simulink model "Demo_TollSystem_cs"  (R2014b)
settings: Solver=FixedStepDiscrete  StartTime=0.0  StopTime=13  FixedStep=1/20  RelTol=1e-3
PreLoadFcn:
  | mbxruntime.callbacks.PreLoadFcn(bdroot);
  | check_NUTS_defined
  | model_closed = 0;
  | assignin('base',['model_closed_' bdroot],false);
PostLoadFcn:
  | mbxruntime.callbacks.PostLoadFcn(bdroot);
InitFcn:
  | mbxruntime.callbacks.InitFcn(bdroot);
StartFcn:
  | mbxruntime.callbacks.StartFcn(bdroot);
  | 
  | open_system([bdroot '/Scope Plot']);
StopFcn:
  | mbxruntime.callbacks.StopFcn(bdroot);
model workspace: external: MAT-File .\Demo_TollSystem_cs_hws.mat (data not in the file)
undefined symbols (not defined in the file): Demo_TollSystem_cs_acfd828c7254e63e, Demo_TollSystem_cs_Mazda_RX8_1_Path_pathUniqueID
libraries: simulink x8, PreScanUsefulBlocks x4
(part 1 of 3)
CloseFcn:
  | mbxruntime.callbacks.CloseFcn(bdroot);
  | evalin('base',['clear model_closed_' bdroot]);
  | model_closed = 1;
settings Model: Creator=PRESCAN  LastModifiedBy=jenkins
settings DataIOCC: SignalLoggingSaveFormat=ModelDataLogs
settings OptimizationCC: InlineParams=on  ExpressionDepthLimit=2147483647  InitFltsAndDblsToZero=on
settings DebuggingCC: SaveWithParameterizedLinksMsg=none  UnderspecifiedInitializationDetection=Classic  MergeDetectMultiDrivingBlocksExec=none  SignalResolutionControl=TryResolveAllWithWarning  SolverPrmCheckMsg=none  MultiTaskDSMMsg=warning  MultiTaskCondExecSysMsg=none  FcnCallInpInsideContextMsg=UseLocalSettings  StateNameClashWarn=warning
settings ModelReferenceCC: UpdateModelReferenceTargets=IfOutOfDate
settings SFSimCC: SimParseCustomCode=off
settings SFSimCC: SimCustomHeaderCode=|
  | #include "prescan.h"
  | #include "prescan_platform.h"
settings RTWCC: IncludeERTFirstTime=on
settings GRTTargetCC: TargetFcnLib=ansi_tfl_tmw.mat  CombineOutputUpdateFcns=off  GRTInterface=on

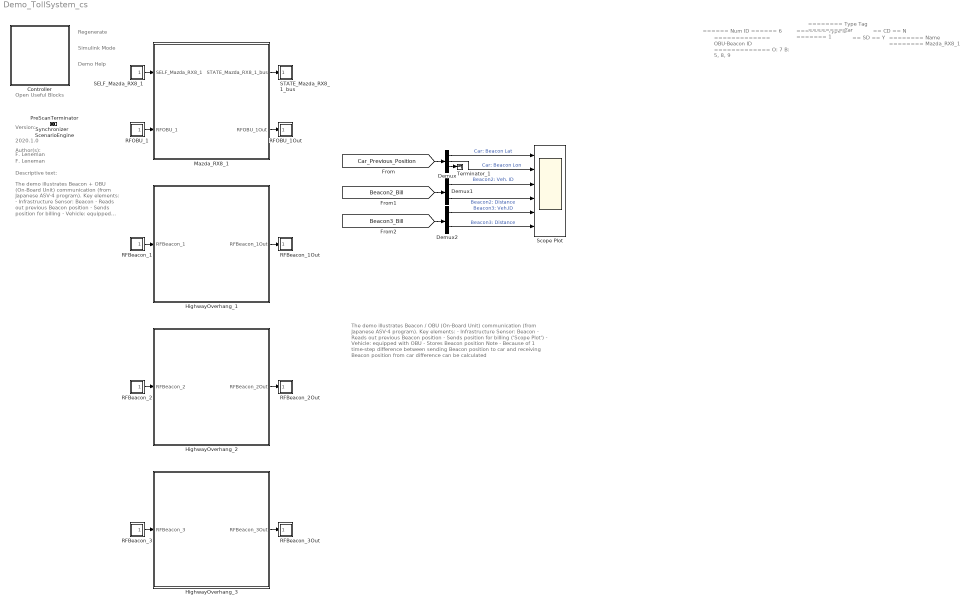
== system Demo_TollSystem_cs ==
  note: Regenerate
  note: Simulink Mode
  note: Open Useful Blocks
  note: 2020.1.0
  note: Version:
  note: Author(s):
  note: F. Leneman
  note: Descriptive text:
  note: The demo illustrates Beacon + OBU
      |
      |
      | (On-Board Unit) communication
      |
      | (from Japanese ASV-4 program).
      |
      |
      |
      | Key elements:
      |
      | - Infrastructure Sensor: Beacon
      |
      |     - Reads out previous Beacon
      | position
      |
      |     - Sends position for billing
      |
      | - Vehicle: equipped with OBU
      |
      |     - Stores Beacon position
  note: The demo illustrates Beacon / OBU (On-Board Unit)
      | communication (from Japanese ASV-4 program).
      |
      | Key elements:
      | - Infrastructure Sensor: Beacon
      |     - Reads out previous Beacon position
      |     - Sends position for billing ('Scope Plot')
      | - Vehicle: equipped with OBU
      |     - Stores Beacon position
      |
      | Note
      | - Because of 1 time-step difference between sending Beacon position
      |   to car and receiving Beacon position from car difference can be
      |   calculated
  note: Demo Help
  note: F. Leneman
  note: ======
      | Num ID
      | ======
      | 6
  note: =============
      | OBU-Beacon ID
      | =============
      | O: 7 B: 5, 8, 9
  note: =======
      | Type ID
      | =======
      | 1
  note: ========
      | Type Tag
      | ========
      | Car
  note: ==
      | SD
      | ==
      | Y
  note: ==
      | CD
      | ==
      | N
  note: ========
      | Name
      | ========
      | Mazda_RX8_1
  Controller : Subsystem  Description=8A3CD2955739A82C886C20AE3E253D78460D53180EE2C1B14CC08DF75A70BE77  Priority=-1  LoadFcn=load PreScanControllerData  mask(PreScan Simulation Controller){prescanversion='2020.1.0', ModelReferencing=off, TimeStep=1/20, ControlMode=0, PreScanExecutionMode=on, ControllerCount=0, ControllerIndex=0, ControllerOptions=''}
      mask prompts: prescanversion "PreScan Version"; ModelReferencing "Use Model Referencing"; TimeStep "Upload Period [s]"; ControlMode "Control Mode"; PreScanExecutionMode "Execution Mode"; ControllerCount "Controller Count"; ControllerIndex "Controller Index"; ControllerOptions "Controller Options"
      mask help:
      | Please do not remove this block from the compilation sheet,
      | as it connects the model to the PreScan environment.
      mask init:
      | model = bdroot(gcb);
      | ExperimentFile = mbxruntime.findExperimentFile(model,true); %relative path
      | 
      | [d1, d2, d3, prescandata] = prescan_Settings();
      | ModelDepo = fullfile(prescandata,'ModelDepo'); 
      | 
      | RTmode = mbxruntime.getRTMode(model);
      | 
      | SimulationMode = get_param(bdroot,'SimulationMode');
      | if strcmp(SimulationMode, 'rapid-accelerator')
      |     SimulationMode = 'external';
      | end
      | TargetName = get_param(bdroot,'SystemTargetFile');
      settings: ModelCloseFcn=assignin('base',['model_closed_' bdroot],true);
      mask Help: eval('openHelp(812)')
      mask Display: image(imread('prescanlogo.ico'))
  Demux : Demux  Outputs=3
  Demux1 : Demux  Outputs=2
  Demux2 : Demux  Outputs=2
  HighwayOverhang_1 : Subsystem  Tag=WorldObjectSubSystem  InitFcn=UniqueId = '39';
      mask init:
      | imagePath=which('HighwayOverhang.jpg');
      mask Display: image(imread(imagePath));color('white');text(0, 0, ' ID=2\n')
  HighwayOverhang_2 : Subsystem  Tag=WorldObjectSubSystem  InitFcn=UniqueId = '40';
      mask init:
      | imagePath=which('HighwayOverhang.jpg');
      mask Display: image(imread(imagePath));color('white');text(0, 0, ' ID=3\n')
  HighwayOverhang_3 : Subsystem  Tag=WorldObjectSubSystem  InitFcn=UniqueId = '41';
      mask init:
      | imagePath=which('HighwayOverhang.jpg');
      mask Display: image(imread(imagePath));color('white');text(0, 0, ' ID=4\n')
  Mazda_RX8_1 : Subsystem  Tag=WorldObjectSubSystem  InitFcn=UniqueId = '16';
      mask init:
      | modelPath = GenericModelHelper.getGenericModelFilePath('ModelDepo','Vehicles\Mazda_RX8\Mazda_RX8.pgmb','1e55a2e40efa576b7f4fb93bae35d605');imagePath = GenericModelHelper.getCompilationPicture(modelPath, 'Mazda_RX8_HighPoly.png');
      mask Display: image(imread(imagePath));color('white');text(0, 0, ' ID=6\n')
  PreScanTerminator : Subsystem  Tag=PreScanTerminator  Priority=999  LoadFcn=load PrescanTerminatorData  mask(PreScan Simulation Terminator){TimeStep=1/20}
      mask prompts: TimeStep "Upload Period [s]"
      mask help:
      | Please do not remove this block from the compilation sheet as it
      | connects the model to the PreScan environment.
      mask Help: eval('openHelp(812)')
      mask Display: image(imread('prescanlogo.ico'))
  RFBeacon_1 : Subsystem  Tag=sensor/BeaconAndOBU/RFBeaconSensor  Priority=30  LoadFcn=load('PrescanBeaconData.mat');load('PrescanBeaconMessage.mat')  mask(PreScan Source Block: RFBeacon I/O){}
      mask help:
      | Using the Beacon and OBU (On-Board Unit) information between actors and infrastructure can be exchanged.
      |
      | The Beacon Receiver receives actor information and user-definable signals.
      |
      | For more information, please click Help.
      settings: OpenFcn=open_system([gcb '/Sensor'],'mask')
      mask Help: eval('openHelp(486)')
      mask Display: image(imread('ico_Beacon_RF_24_gray.png'))
  RFBeacon_1Out : Subsystem  Tag=actuator/BeaconAndOBU/RFBeaconSensor  Priority=0  LoadFcn=load('PrescanBeaconOBUInputData.mat')  mask(PreScan Sink Block: RFBeacon I/O){}
      mask help:
      | Using the Beacon and OBU (On-Board Unit) information between actors and infrastructure can be exchanged.
      |
      | The Beacon Transmitter contains the following, user-definable signals:
      |
      | - Beacon Type		[-]
      | - Spares (1:15)		[-]
      |
      | For more information, please click Help.
      settings: OpenFcn=open_system([gcb '/Actuator'],'mask')
      mask Help: eval('openHelp(486)')
      mask Display: image(imread('ico_Beacon_RF_24_gray.png'))
  RFBeacon_2 : Subsystem  Tag=sensor/BeaconAndOBU/RFBeaconSensor  Priority=30  LoadFcn=load('PrescanBeaconData.mat');load('PrescanBeaconMessage.mat')  mask(PreScan Source Block: RFBeacon I/O){}
      mask help:
      | Using the Beacon and OBU (On-Board Unit) information between actors and infrastructure can be exchanged.
      |
      | The Beacon Receiver receives actor information and user-definable signals.
      |
      | For more information, please click Help.
      settings: OpenFcn=open_system([gcb '/Sensor'],'mask')
      mask Help: eval('openHelp(486)')
      mask Display: image(imread('ico_Beacon_RF_24_gray.png'))
  RFBeacon_2Out : Subsystem  Tag=actuator/BeaconAndOBU/RFBeaconSensor  Priority=0  LoadFcn=load('PrescanBeaconOBUInputData.mat')  mask(PreScan Sink Block: RFBeacon I/O){}
      mask help:
      | Using the Beacon and OBU (On-Board Unit) information between actors and infrastructure can be exchanged.
      |
      | The Beacon Transmitter contains the following, user-definable signals:
      |
      | - Beacon Type		[-]
      | - Spares (1:15)		[-]
      |
      | For more information, please click Help.
      settings: OpenFcn=open_system([gcb '/Actuator'],'mask')
      mask Help: eval('openHelp(486)')
      mask Display: image(imread('ico_Beacon_RF_24_gray.png'))
  RFBeacon_3 : Subsystem  Tag=sensor/BeaconAndOBU/RFBeaconSensor  Priority=30  LoadFcn=load('PrescanBeaconData.mat');load('PrescanBeaconMessage.mat')  mask(PreScan Source Block: RFBeacon I/O){}
      mask help:
      | Using the Beacon and OBU (On-Board Unit) information between actors and infrastructure can be exchanged.
      |
      | The Beacon Receiver receives actor information and user-definable signals.
      |
      | For more information, please click Help.
      settings: OpenFcn=open_system([gcb '/Sensor'],'mask')
      mask Help: eval('openHelp(486)')
      mask Display: image(imread('ico_Beacon_RF_24_gray.png'))
  RFBeacon_3Out : Subsystem  Tag=actuator/BeaconAndOBU/RFBeaconSensor  Priority=0  LoadFcn=load('PrescanBeaconOBUInputData.mat')  mask(PreScan Sink Block: RFBeacon I/O){}
      mask help:
      | Using the Beacon and OBU (On-Board Unit) information between actors and infrastructure can be exchanged.
      |
      | The Beacon Transmitter contains the following, user-definable signals:
      |
      | - Beacon Type		[-]
      | - Spares (1:15)		[-]
      |
      | For more information, please click Help.
      settings: OpenFcn=open_system([gcb '/Actuator'],'mask')
      mask Help: eval('openHelp(486)')
      mask Display: image(imread('ico_Beacon_RF_24_gray.png'))
  RFOBU_1 : Subsystem  Tag=sensor/BeaconAndOBU/RFOBU  Priority=30  LoadFcn=load('PrescanOBUData.mat');load('PrescanOBUMessage.mat')  mask(PreScan Source Block: RFOBU I/O){}
      mask help:
      | Using the Beacon and OBU (On-Board Unit) information between actors and infrastructure can be exchanged.
      |
      | The OBU Receiver receives infrastructure information and user-definable signals.
      |
      | For more information, please click Help.
      settings: OpenFcn=open_system([gcb '/Sensor'],'mask')
      mask Help: eval('openHelp(487)')
      mask Display: image(imread('ico_OBU_RF_24_gray.png'))
  RFOBU_1Out : Subsystem  Tag=actuator/BeaconAndOBU/RFOBU  Priority=0  LoadFcn=load('PrescanBeaconOBUInputData.mat')  mask(PreScan Sink Block: RFOBU I/O){}
      mask help:
      | Using the Beacon and OBU (On-Board Unit) information between actors and infrastructure can be exchanged.
      |
      | The OBU Transmitter contains the following, user-definable signals:
      |
      | - Vehicle Type		[-]
      | - Spares (1:15)		[-]
      |
      | For more information, please click Help.
      settings: OpenFcn=open_system([gcb '/Actuator'],'mask')
      mask Help: eval('openHelp(487)')
      mask Display: image(imread('ico_OBU_RF_24_gray.png'))
  SELF_Mazda_RX8_1 : Subsystem  Tag=sensor/SelfPort  Priority=30  LoadFcn=load('PreScanSelfSensorData.mat')  mask(PreScan Source Block: SELF){}
      mask help:
      | The SELF port shows (state) information of the actor itself. The outputs are position in the experiment's axis system and the GPS coordinates, and the object's absolute velocity and compass heading.
      |
      | For more information, please click Help.
      settings: OpenFcn=open_system([gcb '/Sensor'],'mask')
      mask Help: eval('openHelp(462)')
      mask Display: image(imread('GPS.png'))
  STATE_Mazda_RX8_1_bus : Subsystem  Tag=actuator/StatePort  Priority=0  LoadFcn=load('PreScanStateActuatorData.mat')  mask(PreScan Sink Block: State){}
      mask help:
      | The Actor State contains a vector signal of size (9x1), containing the following signals:
      |
      | -  Position    	(x,y,z)             	[m]
      | -  Velocity    	(vx,vy,vz)         	[m/s]
      | -  Angles       	(Roll, Pitch, Yaw)	[rad]
      |
      | The Actor state is defined in the global axis system.
      | The state is superponed on the Initial position defined in the GUI.
      |
      | For more information, please click Help.
      settings: OpenFcn=open_system([gcb '/Actuator'],'mask')
      mask Help: eval('openHelp(222)')
      mask Display: image(imread('State.png'))
  ScenarioEngine : Subsystem  Tag=PreScanOpenScenarioBlock  Priority=10  LoadFcn=load PrescanSynchronizeData  mask(PreScan Simulation Core Block){TimeStep=1/20}
      mask prompts: TimeStep "Timestep [s]"
      mask help:
      | Please do not remove this block from the PreScan compilation sheet,
      | as it contains essential configuration parameters for a PreScan simulation.
      settings: DeleteFcn=PreScanBlockDeleteFcn;
      mask Display: image(imread('prescanlogo.ico'))
  Scope Plot : Scope  NumInputPorts=6
      settings: TimeRange=14  YMin=50~5~0~0~0~0  YMax=55~5.005~200000000000000~100~200000000000000~100
  Synchronizer : Subsystem  Tag=PreScanSynchronizer  Priority=20  LoadFcn=load PrescanSynchronizeData  mask(PreScan Simulation Core Block){TimeStep=1/20}
      mask prompts: TimeStep "Timestep [s]"
      mask help:
      | Please do not remove this block from the PreScan compilation sheet,
      | as it contains essential configuration parameters for a PreScan simulation.
      settings: DeleteFcn=PreScanBlockDeleteFcn;
      mask Display: image(imread('prescanlogo.ico'))
  Terminator_1 : Terminator
  wires:
  Demux/1 -> Scope Plot/1  "Car: Beacon Lat"
  Demux1/1 -> Scope Plot/3  "Beacon2: Veh. ID"
  Demux1/2 -> Scope Plot/4  "Beacon2: Distance"
  [Beacon2_Bill] -> Demux1/1
  Demux2/1 -> Scope Plot/5  "Beacon3: Veh.ID"
  Demux2/2 -> Scope Plot/6  "Beacon3: Distance"
  [Beacon3_Bill] -> Demux2/1
  Demux/2 -> Scope Plot/2  "Car: Beacon Lon"
  [Car_Previous_Position] -> Demux/1
  Mazda_RX8_1/1(STATE_Mazda_RX8_1_bus) -> STATE_Mazda_RX8_1_bus/1(STATE_Mazda_RX8_1_bus)
  SELF_Mazda_RX8_1/1(SELF_Mazda_RX8_1) -> Mazda_RX8_1/1(SELF_Mazda_RX8_1)
  RFOBU_1/1(RFOBU_1) -> Mazda_RX8_1/2(RFOBU_1)
  Mazda_RX8_1/2(RFOBU_1Out) -> RFOBU_1Out/1(RFOBU_1Out)
  RFBeacon_1/1(RFBeacon_1) -> HighwayOverhang_1/1(RFBeacon_1)
  HighwayOverhang_1/1(RFBeacon_1Out) -> RFBeacon_1Out/1(RFBeacon_1Out)
  RFBeacon_2/1(RFBeacon_2) -> HighwayOverhang_2/1(RFBeacon_2)
  HighwayOverhang_2/1(RFBeacon_2Out) -> RFBeacon_2Out/1(RFBeacon_2Out)
  RFBeacon_3/1(RFBeacon_3) -> HighwayOverhang_3/1(RFBeacon_3)
  HighwayOverhang_3/1(RFBeacon_3Out) -> RFBeacon_3Out/1(RFBeacon_3Out)
  Demux/3 -> Terminator_1/1

== system Demo_TollSystem_cs/Controller ==
  Terminator : Terminator
  sfun_Controller : S-Function  FunctionName=sfun_Controller  Parameters=SParameter1, SParameter2, SParameter3, SParameter4, SParameter5, SParameter6, SParameter7, SParameter8, SParameter9, SParameter10, SampleTime  EnableBusSupport=off  mask(Legacy Function){SFunctionSpec=void prescan_outputFcn(void** work1, PRESCAN_CONTROLLERDATA y1[1]), SParameter1=uint8([ExperimentFile 0]), SParameter2=uint8([ModelDepo 0]), SParameter3=uint8([ControllerOptions 0]), SParameter4=RTmode, SParameter5=PreScanExecutionMode, SParameter6=ControlMode, SParameter7=ControllerCount, SParameter8=ControllerIndex, SParameter9=uint8([SimulationMode 0]), SParameter10=uint8([TargetName 0]), SampleTime=TimeStep, ShowSpec=on}
      mask prompts: SParameter1 "P1:"; SParameter2 "P2:"; SParameter3 "P3:"; SParameter4 "P4:"; SParameter5 "P5:"; SParameter6 "P6:"; SParameter7 "P7:"; SParameter8 "P8:"; SParameter9 "P9:"; SParameter10 "P10:"; SampleTime "Sample time (-1 for inherited):"; ShowSpec "Display function specification"
      mask help:
      | This block allows you to call the legacy functions specified by the following Legacy Code Tool definition:
      | def.SFunctionName = 'sfun_Controller';
      | def.OutputFcnSpec = 'void prescan_outputFcn(void** work1, PRESCAN_CONTROLLERDATA y1[1])';
      | def.StartFcnSpec = 'void prescan_startFcn(void ** work1, uint8 p1[], uint8 p2[], uint8 p3[], double p4, double p5, double p6, double p7, double p8, uint8 p9[], uint8 p10[])';
      | def.TerminateFcnSpec = 'void prescan_terminateFcn(void** work1)';
      | def.HeaderFiles = {'prescan_controller_data.h', 'prescan_SFunLibrary.h', 'prescan_CreateLogHandler.h', 'prescan_CreateErrorHandler.h', 'prescan_modify.h', 'ModuleDLL.h'};
      | def.SourceFiles = {'prescan_MexLogHandler.c', 'prescan_SimStructErrorHandler.c', 'prescan_LogHandler.c', 'prescan_ErrorHandler.c', 'prescan_Modify.c'};
      | def.HostLibFiles = {'sensorinterfaced.lib'};
      | def.TargetLibFiles = {'sensorinterfaced.so'};
      | def.IncPaths = {'.', 'C:\projects\prescan\rt_vislibrary\vis\..\pimp\include\sensors\InterfaceRTW'};
      | def.SrcPaths = {'C:\projects\prescan\rt_vislibrary\vis\..\pimp\include\sensors\InterfaceRTW', 'C:\projects\prescan\rt_vislibrary\vis\..\pimp\include\sensors\InterfaceRTW\ccurrt'};
      | def.LibPaths = {'C:\\projects\\prescan\\vislibrary_build\lib'};
      | def.SampleTime = 'parameterized';
      mask Help: <p>This block was generated automatically by the Legacy Code Tool. For detailed help on this tool, call<a href="matlab:legacy_code('help')"> legacy_code('help')</a>.</p>
      mask Callback ShowSpec:
      | if strcmp(get_param(gcbh, 'ShowSpec'), 'on')
      |   set_param(gcbh, 'MaskDisplay', sprintf('fprintf(''%s'');', get_param(gcbh, 'SFunctionSpec')));
      | else
      |   set_param(gcbh, 'MaskDisplay', sprintf('fprintf(''%s'');', get_param(gcbh, 'FunctionName')));
      | end
      mask Display: fprintf('void prescan_outputFcn(void** work1, PRESCAN_CONTROLLERDATA y1[1])');
  wires:
  sfun_Controller/1 -> Terminator/1

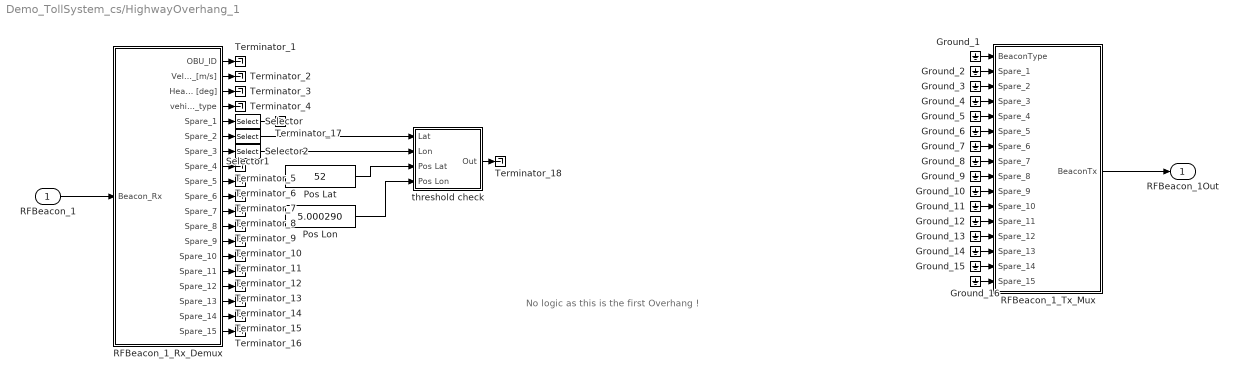
== system Demo_TollSystem_cs/HighwayOverhang_1 ==
  note: No logic as this is the first Overhang !
  RFBeacon_1 : Inport  Tag=inport/BeaconAndOBU/RFBeaconSensor  OutDataTypeStr=Bus: PRESCAN_BEACON_MESSAGE  PortDimensions=5  SampleTime=1/20  BusOutputAsStruct=on
  Ground_{1..16} (16 alike) : Ground
  Pos Lat : Constant  Value=52
  Pos Lon : Constant  Value=5.000290
  RFBeacon_1_Rx_Demux : Subsystem  Tag=demux/BeaconAndOBU  mask(PreScan Demux Block:){Technology='RF', detectableObjects=5}
      mask prompts: detectableObjects "Detectable objects"
      mask init:
      | IconTxt = char('','','','','Technology:            ',['{\it',Technology,'}']);
      settings: DeleteFcn=PreScanBlockDeleteFcn;
      mask Help: eval('openHelp(486)')
      mask Display:
      | disp(IconTxt,'texmode','on')
      | 
      | port_label('output', 1, 'OBU ID [-]')
      | port_label('output', 2, 'OBU Velocity [m/s]')
      | port_label('output', 3, 'OBU Heading [deg]')
      | 
      | port_label('output', 4, 'Vehicle Type [-]')
      | 
      | port_label('output', 5, 'Spare_1')
      | port_label('output', 6, 'Spare_2')
      | port_label('output', 7, 'Spare_3')
      | port_label('output', 8, 'Spare_4')
      | port_label('output', 9, 'Spare_5')
      | 
      | port_label('output', 10, 'Spare_6')
      | port_label('output', 11, 'Spare_7')
      | port_label('output', 12, 'Spare_8')
      | port_label('output', 13, 'Spare_9')
      | port_label('output', 14, 'Spare_10')
      | 
      | port_label('output', 15, 'Spare_11')
      | port_label('output', 16, 'Spare_12')
      | port_label('output', 17, 'Spare_13')
      | port_label('output', 18, 'Spare_14')
      | port_label('output', 19, 'Spare_15')
  RFBeacon_1_Tx_Mux : Subsystem  Tag=mux/BeaconAndOBU_TA/BeaconTx  mask(PreScan Mux Block:){Technology='RF'}
      mask init:
      | IconTxt = char('','','','              Technology:',['{\it                ',Technology,'}']);
      settings: DeleteFcn=PreScanBlockDeleteFcn;
      mask Help: eval('openHelp(486)')
      mask Display:
      | disp(IconTxt,'texmode','on')
      | 
      | port_label('input', 1, 'Beacon Type')
      | 
      | port_label('input', 2, 'Spare_1')
      | port_label('input', 3, 'Spare_2')
      | port_label('input', 4, 'Spare_3')
      | port_label('input', 5, 'Spare_4')
      | port_label('input', 6, 'Spare_5')
      | 
      | port_label('input', 7, 'Spare_6')
      | port_label('input', 8, 'Spare_7')
      | port_label('input', 9, 'Spare_8')
      | port_label('input', 10, 'Spare_9')
      | port_label('input', 11, 'Spare_10')
      | 
      | port_label('input', 12, 'Spare_11')
      | port_label('input', 13, 'Spare_12')
      | port_label('input', 14, 'Spare_13')
      | port_label('input', 15, 'Spare_14')
      | port_label('input', 16, 'Spare_15')
  Selector : Selector  Indices=[1]
  Selector1 : Selector  Indices=[1]
  Selector2 : Selector  Indices=[1]
  Terminator_{1..18} (18 alike) : Terminator
  threshold check : Subsystem
  RFBeacon_1Out : Outport  Tag=outport/BeaconAndOBU/RFBeaconSensor  OutDataTypeStr=Bus: PRESCAN_BEACONOBU_INPUT_DATA  PortDimensions=1  SampleTime=1/20
  wires:
  Pos Lat/1 -> threshold check/3(Pos Lat)
  Selector1/1 -> threshold check/1(Lat)
  Selector2/1 -> threshold check/2(Lon)
  Pos Lon/1 -> threshold check/4(Pos Lon)
  RFBeacon_1_Rx_Demux/6(Spare_2) -> Selector1/1
  RFBeacon_1_Rx_Demux/7(Spare_3) -> Selector2/1
  RFBeacon_1_Rx_Demux/5(Spare_1) -> Selector/1
  RFBeacon_1/1 -> RFBeacon_1_Rx_Demux/1(Beacon_Rx)
  RFBeacon_1_Tx_Mux/1(BeaconTx) -> RFBeacon_1Out/1
  RFBeacon_1_Rx_Demux/1(OBU_ID) -> Terminator_1/1
  RFBeacon_1_Rx_Demux/2(Velocity_[m/s]) -> Terminator_2/1
  RFBeacon_1_Rx_Demux/3(Heading [deg]) -> Terminator_3/1
  RFBeacon_1_Rx_Demux/4(vehicle_type) -> Terminator_4/1
  RFBeacon_1_Rx_Demux/8(Spare_4) -> Terminator_5/1
  RFBeacon_1_Rx_Demux/9(Spare_5) -> Terminator_6/1
  RFBeacon_1_Rx_Demux/10(Spare_6) -> Terminator_7/1
  RFBeacon_1_Rx_Demux/11(Spare_7) -> Terminator_8/1
  RFBeacon_1_Rx_Demux/12(Spare_8) -> Terminator_9/1
  RFBeacon_1_Rx_Demux/13(Spare_9) -> Terminator_10/1
  RFBeacon_1_Rx_Demux/14(Spare_10) -> Terminator_11/1
  RFBeacon_1_Rx_Demux/15(Spare_11) -> Terminator_12/1
  RFBeacon_1_Rx_Demux/16(Spare_12) -> Terminator_13/1
  RFBeacon_1_Rx_Demux/17(Spare_13) -> Terminator_14/1
  RFBeacon_1_Rx_Demux/18(Spare_14) -> Terminator_15/1
  RFBeacon_1_Rx_Demux/19(Spare_15) -> Terminator_16/1
  Ground_1/1 -> RFBeacon_1_Tx_Mux/1(BeaconType)
  Ground_2/1 -> RFBeacon_1_Tx_Mux/2(Spare_1)
  Ground_3/1 -> RFBeacon_1_Tx_Mux/3(Spare_2)
  Ground_4/1 -> RFBeacon_1_Tx_Mux/4(Spare_3)
  Ground_5/1 -> RFBeacon_1_Tx_Mux/5(Spare_4)
  Ground_6/1 -> RFBeacon_1_Tx_Mux/6(Spare_5)
  Ground_7/1 -> RFBeacon_1_Tx_Mux/7(Spare_6)
  Ground_8/1 -> RFBeacon_1_Tx_Mux/8(Spare_7)
  Ground_9/1 -> RFBeacon_1_Tx_Mux/9(Spare_8)
  Ground_10/1 -> RFBeacon_1_Tx_Mux/10(Spare_9)
  Ground_11/1 -> RFBeacon_1_Tx_Mux/11(Spare_10)
  Ground_12/1 -> RFBeacon_1_Tx_Mux/12(Spare_11)
  Ground_13/1 -> RFBeacon_1_Tx_Mux/13(Spare_12)
  Ground_14/1 -> RFBeacon_1_Tx_Mux/14(Spare_13)
  Ground_15/1 -> RFBeacon_1_Tx_Mux/15(Spare_14)
  Ground_16/1 -> RFBeacon_1_Tx_Mux/16(Spare_15)
  Selector/1 -> Terminator_17/1
  threshold check/1(Out) -> Terminator_18/1

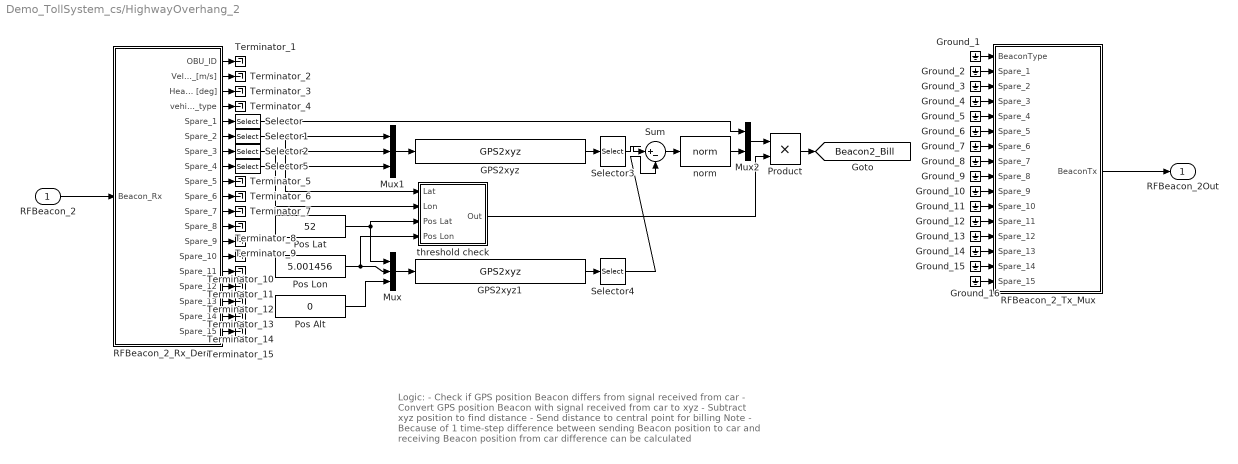
== system Demo_TollSystem_cs/HighwayOverhang_2 ==
  note: Logic:
      | - Check if GPS position Beacon differs from signal received from car
      | - Convert GPS position Beacon with signal received from car to xyz
      | - Subtract xyz position to find distance
      | - Send distance to central point for billing
      |
      | Note
      | - Because of 1 time-step difference between sending Beacon position
      |   to car and receiving Beacon position from car difference can be
      |   calculated
  RFBeacon_2 : Inport  Tag=inport/BeaconAndOBU/RFBeaconSensor  OutDataTypeStr=Bus: PRESCAN_BEACON_MESSAGE  PortDimensions=5  SampleTime=1/20  BusOutputAsStruct=on
  GPS2xyz : PreScanUsefulBlocks/GPS2xyz  CoordinateCount=1  GPS_base=[52 5 0]
  GPS2xyz1 : PreScanUsefulBlocks/GPS2xyz  CoordinateCount=1  GPS_base=[52 5 0]
  Ground_{1..16} (16 alike) : Ground
  Mux : Mux  Inputs=3
  Mux1 : Mux  Inputs=3
  Mux2 : Mux  Inputs=2
  Pos Alt : Constant  Value=0
  Pos Lat : Constant  Value=52
  Pos Lon : Constant  Value=5.001456
  Product : Product  RndMeth=Zero
  RFBeacon_2_Rx_Demux : Subsystem  Tag=demux/BeaconAndOBU  mask(PreScan Demux Block:){Technology='RF', detectableObjects=5}
      mask prompts: detectableObjects "Detectable objects"
      mask init:
      | IconTxt = char('','','','','Technology:            ',['{\it',Technology,'}']);
      settings: DeleteFcn=PreScanBlockDeleteFcn;
      mask Help: eval('openHelp(486)')
      mask Display:
      | disp(IconTxt,'texmode','on')
      | 
      | port_label('output', 1, 'OBU ID [-]')
      | port_label('output', 2, 'OBU Velocity [m/s]')
      | port_label('output', 3, 'OBU Heading [deg]')
      | 
      | port_label('output', 4, 'Vehicle Type [-]')
      | 
      | port_label('output', 5, 'Spare_1')
      | port_label('output', 6, 'Spare_2')
      | port_label('output', 7, 'Spare_3')
      | port_label('output', 8, 'Spare_4')
      | port_label('output', 9, 'Spare_5')
      | 
      | port_label('output', 10, 'Spare_6')
      | port_label('output', 11, 'Spare_7')
      | port_label('output', 12, 'Spare_8')
      | port_label('output', 13, 'Spare_9')
      | port_label('output', 14, 'Spare_10')
      | 
      | port_label('output', 15, 'Spare_11')
      | port_label('output', 16, 'Spare_12')
      | port_label('output', 17, 'Spare_13')
      | port_label('output', 18, 'Spare_14')
      | port_label('output', 19, 'Spare_15')
  RFBeacon_2_Tx_Mux : Subsystem  Tag=mux/BeaconAndOBU_TA/BeaconTx  mask(PreScan Mux Block:){Technology='RF'}
      mask init:
      | IconTxt = char('','','','              Technology:',['{\it                ',Technology,'}']);
      settings: DeleteFcn=PreScanBlockDeleteFcn;
      mask Help: eval('openHelp(486)')
      mask Display:
      | disp(IconTxt,'texmode','on')
      | 
      | port_label('input', 1, 'Beacon Type')
      | 
      | port_label('input', 2, 'Spare_1')
      | port_label('input', 3, 'Spare_2')
      | port_label('input', 4, 'Spare_3')
      | port_label('input', 5, 'Spare_4')
      | port_label('input', 6, 'Spare_5')
      | 
      | port_label('input', 7, 'Spare_6')
      | port_label('input', 8, 'Spare_7')
      | port_label('input', 9, 'Spare_8')
      | port_label('input', 10, 'Spare_9')
      | port_label('input', 11, 'Spare_10')
      | 
      | port_label('input', 12, 'Spare_11')
      | port_label('input', 13, 'Spare_12')
      | port_label('input', 14, 'Spare_13')
      | port_label('input', 15, 'Spare_14')
      | port_label('input', 16, 'Spare_15')
  Selector{,1..2,5} (4 alike) : Selector  Indices=[1]
  Selector3 : Selector  InputPortWidth=3  Indices=[1 2]
  Selector4 : Selector  InputPortWidth=3  Indices=[1 2]
  Sum : Sum  Inputs=|+-
  Terminator_{1..15} (15 alike) : Terminator
  norm : MATLABFcn  MATLABFcn=norm
  threshold check : Subsystem
  RFBeacon_2Out : Outport  Tag=outport/BeaconAndOBU/RFBeaconSensor  OutDataTypeStr=Bus: PRESCAN_BEACONOBU_INPUT_DATA  PortDimensions=1  SampleTime=1/20
  tag scope: Beacon2_Bill=global
  wires:
  GPS2xyz/1 -> Selector3/1
  Selector3/1 -> Sum/1
  Sum/1 -> norm/1
  norm/1 -> Mux2/2
  Mux2/1 -> Product/1
  Product/1 -> [Beacon2_Bill]
  threshold check/1(Out) -> Product/2
  Selector1/1 -> threshold check/1(Lat), Mux1/1
  Mux1/1 -> GPS2xyz/1
  Selector2/1 -> Mux1/2, threshold check/2(Lon)
  Selector5/1 -> Mux1/3
  Pos Lat/1 -> threshold check/3(Pos Lat), Mux/1
  Mux/1 -> GPS2xyz1/1
  GPS2xyz1/1 -> Selector4/1
  Selector4/1 -> Sum/2
  Pos Lon/1 -> threshold check/4(Pos Lon), Mux/2
  Pos Alt/1 -> Mux/3
  Selector/1 -> Mux2/1
  RFBeacon_2_Rx_Demux/7(Spare_3) -> Selector2/1
  RFBeacon_2_Rx_Demux/8(Spare_4) -> Selector5/1
  RFBeacon_2_Rx_Demux/6(Spare_2) -> Selector1/1
  RFBeacon_2_Rx_Demux/5(Spare_1) -> Selector/1
  RFBeacon_2/1 -> RFBeacon_2_Rx_Demux/1(Beacon_Rx)
  RFBeacon_2_Tx_Mux/1(BeaconTx) -> RFBeacon_2Out/1
  RFBeacon_2_Rx_Demux/1(OBU_ID) -> Terminator_1/1
  RFBeacon_2_Rx_Demux/2(Velocity_[m/s]) -> Terminator_2/1
  RFBeacon_2_Rx_Demux/3(Heading [deg]) -> Terminator_3/1
  RFBeacon_2_Rx_Demux/4(vehicle_type) -> Terminator_4/1
  RFBeacon_2_Rx_Demux/9(Spare_5) -> Terminator_5/1
  RFBeacon_2_Rx_Demux/10(Spare_6) -> Terminator_6/1
  RFBeacon_2_Rx_Demux/11(Spare_7) -> Terminator_7/1
  RFBeacon_2_Rx_Demux/12(Spare_8) -> Terminator_8/1
  RFBeacon_2_Rx_Demux/13(Spare_9) -> Terminator_9/1
  RFBeacon_2_Rx_Demux/14(Spare_10) -> Terminator_10/1
  RFBeacon_2_Rx_Demux/15(Spare_11) -> Terminator_11/1
  RFBeacon_2_Rx_Demux/16(Spare_12) -> Terminator_12/1
  RFBeacon_2_Rx_Demux/17(Spare_13) -> Terminator_13/1
  RFBeacon_2_Rx_Demux/18(Spare_14) -> Terminator_14/1
  RFBeacon_2_Rx_Demux/19(Spare_15) -> Terminator_15/1
  Ground_1/1 -> RFBeacon_2_Tx_Mux/1(BeaconType)
  Ground_2/1 -> RFBeacon_2_Tx_Mux/2(Spare_1)
  Ground_3/1 -> RFBeacon_2_Tx_Mux/3(Spare_2)
  Ground_4/1 -> RFBeacon_2_Tx_Mux/4(Spare_3)
  Ground_5/1 -> RFBeacon_2_Tx_Mux/5(Spare_4)
  Ground_6/1 -> RFBeacon_2_Tx_Mux/6(Spare_5)
  Ground_7/1 -> RFBeacon_2_Tx_Mux/7(Spare_6)
  Ground_8/1 -> RFBeacon_2_Tx_Mux/8(Spare_7)
  Ground_9/1 -> RFBeacon_2_Tx_Mux/9(Spare_8)
  Ground_10/1 -> RFBeacon_2_Tx_Mux/10(Spare_9)
  Ground_11/1 -> RFBeacon_2_Tx_Mux/11(Spare_10)
  Ground_12/1 -> RFBeacon_2_Tx_Mux/12(Spare_11)
  Ground_13/1 -> RFBeacon_2_Tx_Mux/13(Spare_12)
  Ground_14/1 -> RFBeacon_2_Tx_Mux/14(Spare_13)
  Ground_15/1 -> RFBeacon_2_Tx_Mux/15(Spare_14)
  Ground_16/1 -> RFBeacon_2_Tx_Mux/16(Spare_15)

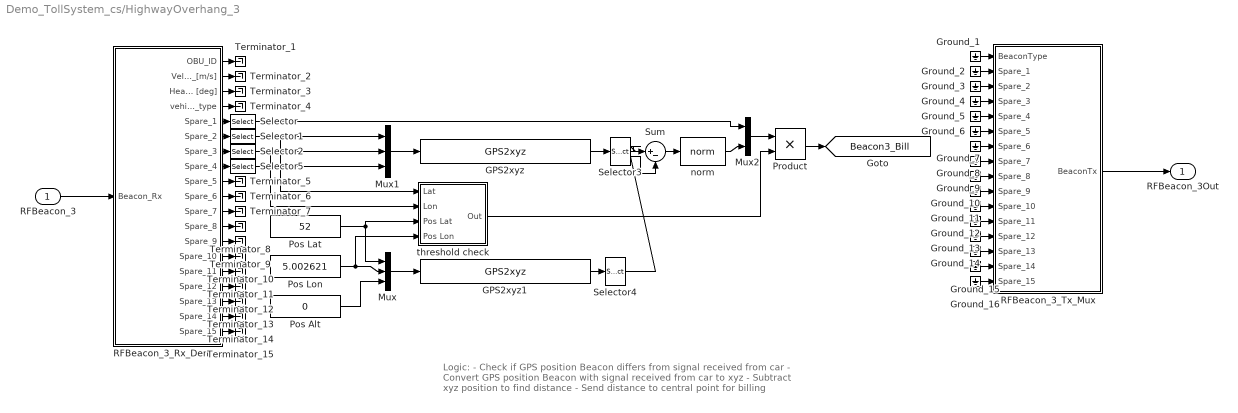
== system Demo_TollSystem_cs/HighwayOverhang_3 ==
  note: Logic:
      | - Check if GPS position Beacon differs from signal received from car
      | - Convert GPS position Beacon with signal received from car to xyz
      | - Subtract xyz position to find distance
      | - Send distance to central point for billing
  RFBeacon_3 : Inport  Tag=inport/BeaconAndOBU/RFBeaconSensor  OutDataTypeStr=Bus: PRESCAN_BEACON_MESSAGE  PortDimensions=5  SampleTime=1/20  BusOutputAsStruct=on
  GPS2xyz : PreScanUsefulBlocks/GPS2xyz  CoordinateCount=1  GPS_base=[52 5 0]
  GPS2xyz1 : PreScanUsefulBlocks/GPS2xyz  CoordinateCount=1  GPS_base=[52 5 0]
  Ground_{1..16} (16 alike) : Ground
  Mux : Mux  Inputs=3
  Mux1 : Mux  Inputs=3
  Mux2 : Mux  Inputs=2
  Pos Alt : Constant  Value=0
  Pos Lat : Constant  Value=52
  Pos Lon : Constant  Value=5.002621
  Product : Product  RndMeth=Zero
  RFBeacon_3_Rx_Demux : Subsystem  Tag=demux/BeaconAndOBU  mask(PreScan Demux Block:){Technology='RF', detectableObjects=5}
      mask prompts: detectableObjects "Detectable objects"
      mask init:
      | IconTxt = char('','','','','Technology:            ',['{\it',Technology,'}']);
      settings: DeleteFcn=PreScanBlockDeleteFcn;
      mask Help: eval('openHelp(486)')
      mask Display:
      | disp(IconTxt,'texmode','on')
      | 
      | port_label('output', 1, 'OBU ID [-]')
      | port_label('output', 2, 'OBU Velocity [m/s]')
      | port_label('output', 3, 'OBU Heading [deg]')
      | 
      | port_label('output', 4, 'Vehicle Type [-]')
      | 
      | port_label('output', 5, 'Spare_1')
      | port_label('output', 6, 'Spare_2')
      | port_label('output', 7, 'Spare_3')
      | port_label('output', 8, 'Spare_4')
      | port_label('output', 9, 'Spare_5')
      | 
      | port_label('output', 10, 'Spare_6')
      | port_label('output', 11, 'Spare_7')
      | port_label('output', 12, 'Spare_8')
      | port_label('output', 13, 'Spare_9')
      | port_label('output', 14, 'Spare_10')
      | 
      | port_label('output', 15, 'Spare_11')
      | port_label('output', 16, 'Spare_12')
      | port_label('output', 17, 'Spare_13')
      | port_label('output', 18, 'Spare_14')
      | port_label('output', 19, 'Spare_15')
  RFBeacon_3_Tx_Mux : Subsystem  Tag=mux/BeaconAndOBU_TA/BeaconTx  mask(PreScan Mux Block:){Technology='RF'}
      mask init:
      | IconTxt = char('','','','              Technology:',['{\it                ',Technology,'}']);
      settings: DeleteFcn=PreScanBlockDeleteFcn;
      mask Help: eval('openHelp(486)')
      mask Display:
      | disp(IconTxt,'texmode','on')
      | 
      | port_label('input', 1, 'Beacon Type')
      | 
      | port_label('input', 2, 'Spare_1')
      | port_label('input', 3, 'Spare_2')
      | port_label('input', 4, 'Spare_3')
      | port_label('input', 5, 'Spare_4')
      | port_label('input', 6, 'Spare_5')
      | 
      | port_label('input', 7, 'Spare_6')
      | port_label('input', 8, 'Spare_7')
      | port_label('input', 9, 'Spare_8')
      | port_label('input', 10, 'Spare_9')
      | port_label('input', 11, 'Spare_10')
      | 
      | port_label('input', 12, 'Spare_11')
      | port_label('input', 13, 'Spare_12')
      | port_label('input', 14, 'Spare_13')
      | port_label('input', 15, 'Spare_14')
      | port_label('input', 16, 'Spare_15')
  Selector{,1..2,5} (4 alike) : Selector  Indices=[1]
  Selector3 : Selector  InputPortWidth=3  Indices=[1 2]
  Selector4 : Selector  InputPortWidth=3  Indices=[1 2]
  Sum : Sum  Inputs=|+-
  Terminator_{1..15} (15 alike) : Terminator
  norm : MATLABFcn  MATLABFcn=norm
  threshold check : Subsystem
  RFBeacon_3Out : Outport  Tag=outport/BeaconAndOBU/RFBeaconSensor  OutDataTypeStr=Bus: PRESCAN_BEACONOBU_INPUT_DATA  PortDimensions=1  SampleTime=1/20
  tag scope: Beacon3_Bill=global
  wires:
  GPS2xyz/1 -> Selector3/1
  Selector3/1 -> Sum/1
  Sum/1 -> norm/1
  norm/1 -> Mux2/2
  Mux2/1 -> Product/1
  Product/1 -> [Beacon3_Bill]
  threshold check/1(Out) -> Product/2
  Selector1/1 -> threshold check/1(Lat), Mux1/1
  Mux1/1 -> GPS2xyz/1
  Selector2/1 -> Mux1/2, threshold check/2(Lon)
  Selector5/1 -> Mux1/3
  Pos Lat/1 -> threshold check/3(Pos Lat), Mux/1
  Mux/1 -> GPS2xyz1/1
  GPS2xyz1/1 -> Selector4/1
  Selector4/1 -> Sum/2
  Pos Lon/1 -> threshold check/4(Pos Lon), Mux/2
  Pos Alt/1 -> Mux/3
  Selector/1 -> Mux2/1
  RFBeacon_3_Rx_Demux/7(Spare_3) -> Selector2/1
  RFBeacon_3_Rx_Demux/8(Spare_4) -> Selector5/1
  RFBeacon_3_Rx_Demux/6(Spare_2) -> Selector1/1
  RFBeacon_3_Rx_Demux/5(Spare_1) -> Selector/1
  RFBeacon_3/1 -> RFBeacon_3_Rx_Demux/1(Beacon_Rx)
  RFBeacon_3_Tx_Mux/1(BeaconTx) -> RFBeacon_3Out/1
  RFBeacon_3_Rx_Demux/1(OBU_ID) -> Terminator_1/1
  RFBeacon_3_Rx_Demux/2(Velocity_[m/s]) -> Terminator_2/1
  RFBeacon_3_Rx_Demux/3(Heading [deg]) -> Terminator_3/1
  RFBeacon_3_Rx_Demux/4(vehicle_type) -> Terminator_4/1
  RFBeacon_3_Rx_Demux/9(Spare_5) -> Terminator_5/1
  RFBeacon_3_Rx_Demux/10(Spare_6) -> Terminator_6/1
  RFBeacon_3_Rx_Demux/11(Spare_7) -> Terminator_7/1
  RFBeacon_3_Rx_Demux/12(Spare_8) -> Terminator_8/1
  RFBeacon_3_Rx_Demux/13(Spare_9) -> Terminator_9/1
  RFBeacon_3_Rx_Demux/14(Spare_10) -> Terminator_10/1
  RFBeacon_3_Rx_Demux/15(Spare_11) -> Terminator_11/1
  RFBeacon_3_Rx_Demux/16(Spare_12) -> Terminator_12/1
  RFBeacon_3_Rx_Demux/17(Spare_13) -> Terminator_13/1
  RFBeacon_3_Rx_Demux/18(Spare_14) -> Terminator_14/1
  RFBeacon_3_Rx_Demux/19(Spare_15) -> Terminator_15/1
  Ground_1/1 -> RFBeacon_3_Tx_Mux/1(BeaconType)
  Ground_2/1 -> RFBeacon_3_Tx_Mux/2(Spare_1)
  Ground_3/1 -> RFBeacon_3_Tx_Mux/3(Spare_2)
  Ground_4/1 -> RFBeacon_3_Tx_Mux/4(Spare_3)
  Ground_5/1 -> RFBeacon_3_Tx_Mux/5(Spare_4)
  Ground_6/1 -> RFBeacon_3_Tx_Mux/6(Spare_5)
  Ground_7/1 -> RFBeacon_3_Tx_Mux/7(Spare_6)
  Ground_8/1 -> RFBeacon_3_Tx_Mux/8(Spare_7)
  Ground_9/1 -> RFBeacon_3_Tx_Mux/9(Spare_8)
  Ground_10/1 -> RFBeacon_3_Tx_Mux/10(Spare_9)
  Ground_11/1 -> RFBeacon_3_Tx_Mux/11(Spare_10)
  Ground_12/1 -> RFBeacon_3_Tx_Mux/12(Spare_11)
  Ground_13/1 -> RFBeacon_3_Tx_Mux/13(Spare_12)
  Ground_14/1 -> RFBeacon_3_Tx_Mux/14(Spare_13)
  Ground_15/1 -> RFBeacon_3_Tx_Mux/15(Spare_14)
  Ground_16/1 -> RFBeacon_3_Tx_Mux/16(Spare_15)

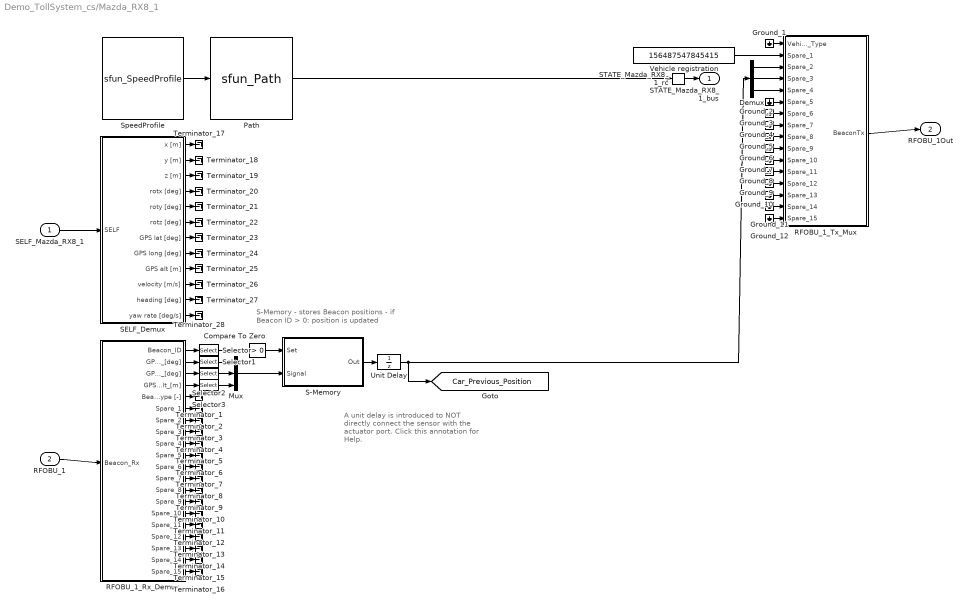
== system Demo_TollSystem_cs/Mazda_RX8_1 ==
  note: A unit delay is introduced to NOT
      | directly connect the sensor with
      | the actuator port.
      |
      | Click this annotation for Help.
  note: S-Memory
      | - stores Beacon positions
      | - if Beacon ID > 0: position is updated
  SELF_Mazda_RX8_1 : Inport  Tag=inport/SelfPort  OutDataTypeStr=Bus: PRESCAN_SELFSENSORDATA  PortDimensions=1  SampleTime=1/20  BusOutputAsStruct=on
  RFOBU_1 : Inport  Tag=inport/BeaconAndOBU/RFOBU  Port=2  OutDataTypeStr=Bus: PRESCAN_OBU_MESSAGE  PortDimensions=2  SampleTime=1/20  BusOutputAsStruct=on
  Compare To Zero : simulink/Logic and Bit Operations/Compare To Zero  relop=>  OutDataTypeStr=uint8  ZeroCross=off
  Demux : Demux  Outputs=3
  Ground_{1..12} (12 alike) : Ground
  Mux : Mux  Inputs=3
  Path : S-Function  Tag=Path  LoadFcn=load('PrescanMotionData.mat')  FunctionName=sfun_Path  Parameters=uniqueID, pathUniqueID, timestep  EnableBusSupport=off  mask(Path){uniqueID=16, pathUniqueID=Demo_TollSystem_cs_Mazda_RX8_1_Path_pathUniqueID, timestep=1/20}
      mask prompts: uniqueID "Object Unique ID"; pathUniqueID "Path Unique ID"; timestep "MATLAB timestep:"
      mask help:
      | The path block outputs the position along a given trajectory.
      |
      | For more information, please click Help.
      mask Help: eval('openHelp(312)')
      mask Display: image(imread('Path.png'))
  RFOBU_1_Rx_Demux : Subsystem  Tag=demux/OBURx  mask(PreScan Demux Block:){Technology='RF', detectableObjects=2}
      mask prompts: detectableObjects "Detectable objects"
      mask init:
      | IconTxt = char('','','','Technology:            ',['{\it',Technology,'}']);
      settings: DeleteFcn=PreScanBlockDeleteFcn;
      mask Help: eval('openHelp(487)')
      mask Display:
      | disp(IconTxt,'texmode','on')
      | 
      | port_label('output', 1, 'Beacon ID [-]')
      | port_label('output', 2, 'Beacon GPS Lat [deg]')
      | port_label('output', 3, 'Beacon GPS Lon [deg]')
      | port_label('output', 4, 'Beacon GPS Alt [m]')
      | port_label('output', 5, 'Beacon Type [-]')
      | 
      | port_label('output', 6, 'Spare_1')
      | port_label('output', 7, 'Spare_2')
      | port_label('output', 8, 'Spare_3')
      | port_label('output', 9, 'Spare_4')
      | port_label('output', 10, 'Spare_5')
      | 
      | port_label('output', 11, 'Spare_6')
      | port_label('output', 12, 'Spare_7')
      | port_label('output', 13, 'Spare_8')
      | port_label('output', 14, 'Spare_9')
      | port_label('output', 15, 'Spare_10')
      | 
      | port_label('output', 16, 'Spare_11')
      | port_label('output', 17, 'Spare_12')
      | port_label('output', 18, 'Spare_13')
      | port_label('output', 19, 'Spare_14')
      | port_label('output', 20, 'Spare_15')
  RFOBU_1_Tx_Mux : Subsystem  Tag=mux/BeaconAndOBU_TA  mask(PreScan Mux Block:){Technology='RF'}
      mask init:
      | IconTxt = char('','','              Technology:',['{\it                ',Technology,'}']);
      settings: DeleteFcn=PreScanBlockDeleteFcn;
      mask Help: eval('openHelp(487)')
      mask Display:
      | disp(IconTxt,'texmode','on')
      | 
      | port_label('input', 1, 'Vehicle Type')
      | 
      | port_label('input', 2, 'Spare_1')
      | port_label('input', 3, 'Spare_2')
      | port_label('input', 4, 'Spare_3')
      | port_label('input', 5, 'Spare_4')
      | port_label('input', 6, 'Spare_5')
      | 
      | port_label('input', 7, 'Spare_6')
      | port_label('input', 8, 'Spare_7')
      | port_label('input', 9, 'Spare_8')
      | port_label('input', 10, 'Spare_9')
      | port_label('input', 11, 'Spare_10')
      | 
      | port_label('input', 12, 'Spare_11')
      | port_label('input', 13, 'Spare_12')
      | port_label('input', 14, 'Spare_13')
      | port_label('input', 15, 'Spare_14')
      | port_label('input', 16, 'Spare_15')
  S-Memory : Subsystem
  SELF_Demux : Subsystem  Tag=demux/SelfPort  mask(PreScan Demux Block:){}
      mask help:
      | The SELF port shows (state) information of the actor itself. The outputs are position in the experiment's axis system and the GPS coordinates, and the object's absolute velocity and compass heading.
      |
      | For more information, please click Help.
      settings: DeleteFcn=PreScanBlockDeleteFcn;
      mask Help: eval('openHelp(462)')
      mask Display:
      | port_label('output',1,'x [m]')
      | port_label('output',2,'y [m]')
      | port_label('output',3,'z [m]','texmode','on')
      | port_label('output',4,'Rotx [deg]','texmode','on')
      | port_label('output',5,'Roty [deg]','texmode','on')
      | port_label('output',6,'Rotz [deg]','texmode','on')
      | port_label('output',7,'GPS lat [deg]','texmode','on')
      | port_label('output',8,'GPS long [deg]','texmode','on')
      | port_label('output',9,'GPS alt [m]','texmode','on')
      | port_label('output',10,'Velocity [m/s]')
      | port_label('output',11,'Heading [deg]')
      | port_label('output',12,'Yaw rate [deg/s]')
  STATE_Mazda_RX8_1_rc : RateTransition  Tag=mux_rc/StatePort  OutPortSampleTimeOpt=Inherit
  Selector{,1..3} (4 alike) : Selector  Indices=[1]
  SpeedProfile : S-Function  Tag=SpeedProfile  LoadFcn=load('PrescanMotionData.mat')  FunctionName=sfun_SpeedProfile  Parameters=speedProfileUniqueID, timestep  EnableBusSupport=off  mask(SpeedProfile){speedProfileUniqueID=Demo_TollSystem_cs_acfd828c7254e63e, timestep=1/20}
      mask prompts: speedProfileUniqueID "Speed Profile Unique ID"; timestep "MATLAB timestep:"
      mask help:
      | The speed profile block outputs the travelled distance, velocities and acceleration along a given path.
      |
      | For more information, please click Help.
      mask Help: eval('openHelp(312)')
      mask Display: image(imread('SpeedProfile.png'))
  Terminator_{1..28} (28 alike) : Terminator
  Unit Delay : UnitDelay  SampleTime=-1
  Vehicle registration : Constant  Value=156487547845415
  STATE_Mazda_RX8_1_bus : Outport  Tag=outport/StatePort  OutDataTypeStr=Bus: PRESCAN_STATEACTUATORDATA  PortDimensions=1  SampleTime=1/20
  RFOBU_1Out : Outport  Tag=outport/BeaconAndOBU/RFOBU  Port=2  OutDataTypeStr=Bus: PRESCAN_BEACONOBU_INPUT_DATA  PortDimensions=1  SampleTime=1/20
  tag scope: Car_Previous_Position=global
  wires:
  Compare To Zero/1 -> S-Memory/1(Set)
  S-Memory/1(Out) -> Unit Delay/1
  Unit Delay/1 -> Demux/1, [Car_Previous_Position]
  Mux/1 -> S-Memory/2(Signal)
  Selector1/1 -> Mux/1
  Selector2/1 -> Mux/2
  Selector3/1 -> Mux/3
  Selector/1 -> Compare To Zero/1
  Demux/1 -> RFOBU_1_Tx_Mux/3(Spare_2)
  Demux/2 -> RFOBU_1_Tx_Mux/4(Spare_3)
  Demux/3 -> RFOBU_1_Tx_Mux/5(Spare_4)
  RFOBU_1_Rx_Demux/2(GPS_pos_lat_[deg]) -> Selector1/1
  RFOBU_1_Rx_Demux/3(GPS_pos_long_[deg]) -> Selector2/1
  RFOBU_1_Rx_Demux/4(GPS_pos_alt_[m]) -> Selector3/1
  RFOBU_1_Rx_Demux/1(Beacon_ID) -> Selector/1
  Vehicle registration/1 -> RFOBU_1_Tx_Mux/2(Spare_1)
  STATE_Mazda_RX8_1_rc/1 -> STATE_Mazda_RX8_1_bus/1
  SpeedProfile/1 -> Path/1
  Path/1 -> STATE_Mazda_RX8_1_rc/1
  SELF_Mazda_RX8_1/1 -> SELF_Demux/1(SELF)
  RFOBU_1/1 -> RFOBU_1_Rx_Demux/1(Beacon_Rx)
  RFOBU_1_Tx_Mux/1(BeaconTx) -> RFOBU_1Out/1
  RFOBU_1_Rx_Demux/5(BeaconType [-]) -> Terminator_1/1
  RFOBU_1_Rx_Demux/6(Spare_1) -> Terminator_2/1
  RFOBU_1_Rx_Demux/7(Spare_2) -> Terminator_3/1
  RFOBU_1_Rx_Demux/8(Spare_3) -> Terminator_4/1
  RFOBU_1_Rx_Demux/9(Spare_4) -> Terminator_5/1
  RFOBU_1_Rx_Demux/10(Spare_5) -> Terminator_6/1
  RFOBU_1_Rx_Demux/11(Spare_6) -> Terminator_7/1
  RFOBU_1_Rx_Demux/12(Spare_7) -> Terminator_8/1
  RFOBU_1_Rx_Demux/13(Spare_8) -> Terminator_9/1
  RFOBU_1_Rx_Demux/14(Spare_9) -> Terminator_10/1
  RFOBU_1_Rx_Demux/15(Spare_10) -> Terminator_11/1
  RFOBU_1_Rx_Demux/16(Spare_11) -> Terminator_12/1
  RFOBU_1_Rx_Demux/17(Spare_12) -> Terminator_13/1
  RFOBU_1_Rx_Demux/18(Spare_13) -> Terminator_14/1
  RFOBU_1_Rx_Demux/19(Spare_14) -> Terminator_15/1
  RFOBU_1_Rx_Demux/20(Spare_15) -> Terminator_16/1
  Ground_1/1 -> RFOBU_1_Tx_Mux/1(Vehicle_Type)
  Ground_2/1 -> RFOBU_1_Tx_Mux/6(Spare_5)
  Ground_3/1 -> RFOBU_1_Tx_Mux/7(Spare_6)
  Ground_4/1 -> RFOBU_1_Tx_Mux/8(Spare_7)
  Ground_5/1 -> RFOBU_1_Tx_Mux/9(Spare_8)
  Ground_6/1 -> RFOBU_1_Tx_Mux/10(Spare_9)
  Ground_7/1 -> RFOBU_1_Tx_Mux/11(Spare_10)
  Ground_8/1 -> RFOBU_1_Tx_Mux/12(Spare_11)
  Ground_9/1 -> RFOBU_1_Tx_Mux/13(Spare_12)
  Ground_10/1 -> RFOBU_1_Tx_Mux/14(Spare_13)
  Ground_11/1 -> RFOBU_1_Tx_Mux/15(Spare_14)
  Ground_12/1 -> RFOBU_1_Tx_Mux/16(Spare_15)
  SELF_Demux/1(x [m]) -> Terminator_17/1
  SELF_Demux/2(y [m]) -> Terminator_18/1
  SELF_Demux/3(z [m]) -> Terminator_19/1
  SELF_Demux/4(rotx [deg]) -> Terminator_20/1
  SELF_Demux/5(roty [deg]) -> Terminator_21/1
  SELF_Demux/6(rotz [deg]) -> Terminator_22/1
  SELF_Demux/7(GPS lat [deg]) -> Terminator_23/1
  SELF_Demux/8(GPS long [deg]) -> Terminator_24/1
  SELF_Demux/9(GPS alt [m]) -> Terminator_25/1
  SELF_Demux/10(velocity [m/s]) -> Terminator_26/1
  SELF_Demux/11(heading [deg]) -> Terminator_27/1
  SELF_Demux/12(yaw rate [deg/s]) -> Terminator_28/1

== system Demo_TollSystem_cs/PreScanTerminator ==
  Terminator : Terminator
  sfun_Terminator : S-Function  FunctionName=sfun_Terminator  Parameters=SampleTime  EnableBusSupport=off  mask(Legacy Function){SFunctionSpec=void prescan_terminator_outputFcn(void ** work1, PRESCAN_TERMINATORDATA y1[1]), SampleTime=TimeStep, ShowSpec=on}
      mask prompts: SampleTime "Sample time (-1 for inherited):"; ShowSpec "Display function specification"
      mask help:
      | This block allows you to call the legacy functions specified by the following Legacy Code Tool definition:
      | def.SFunctionName = 'sfun_Terminator';
      | def.OutputFcnSpec = 'void prescan_terminator_outputFcn(void ** work1, PRESCAN_TERMINATORDATA y1[1])';
      | def.StartFcnSpec = 'void prescan_terminator_startFcn(void ** work1)';
      | def.TerminateFcnSpec = 'void prescan_terminator_terminateFcn(void ** work1)';
      | def.HeaderFiles = {'prescan_terminator_data.h'};
      | def.HostLibFiles = {'sensorinterfaced.lib'};
      | def.IncPaths = {'src', 'C:\prescandev\vislibrary\vis\..\pimp\include\sensors\InterfaceRTW'};
      | def.SrcPaths = {'src'};
      | def.LibPaths = {'C:\\prescandev\\vislibrary_build\lib'};
      | def.SampleTime = 'parameterized';
      | def.Options.language = 'C';
      mask Help: <p>This block was generated automatically by the Legacy Code Tool. For detailed help on this tool, call<a href="matlab:legacy_code('help')"> legacy_code('help')</a>.</p>
      mask Callback ShowSpec:
      | if strcmp(get_param(gcbh, 'ShowSpec'), 'on')
      |   set_param(gcbh, 'MaskDisplay', sprintf('fprintf(''%s'');', get_param(gcbh, 'SFunctionSpec')));
      | else
      |   set_param(gcbh, 'MaskDisplay', sprintf('fprintf(''%s'');', get_param(gcbh, 'FunctionName')));
      | end
      mask Display: fprintf('void prescan_terminator_outputFcn(void ** work1, PRESCAN_TERMINATORDATA y1[1])');
  wires:
  sfun_Terminator/1 -> Terminator/1

== system Demo_TollSystem_cs/RFBeacon_1 ==
  Sensor : S-Function  FunctionName=sfun_Beacon  Parameters=sensorID, NrEntitiesOut, timestep  EnableBusSupport=off  mask(PreScan Source Block: RFBeacon I/O){sensorID=42, NrEntitiesOut=5, timestep=1/20}
      mask prompts: sensorID "Sensor ID"; NrEntitiesOut "User Specified: # of Visible OBUs"; timestep "MATLAB timestep:"
      mask help:
      | Using the Beacon and OBU (On-Board Unit) information between actors and infrastructure can be exchanged.
      |
      | The Beacon Receiver receives actor information and user-definable signals.
      |
      | For more information, please click Help.
      mask Help: eval('openHelp(486)')
      mask Display: image(imread('ico_Beacon_RF_24_gray.png'))
  RFBeacon_1 : Outport  Tag=outport/BeaconAndOBU/RFBeaconSensor  OutDataTypeStr=Bus: PRESCAN_BEACON_MESSAGE  PortDimensions=5  SampleTime=1/20
  wires:
  Sensor/1 -> RFBeacon_1/1

== system Demo_TollSystem_cs/RFBeacon_1Out ==
  RFBeacon_1Out : Inport  Tag=inport/BeaconAndOBU/RFBeaconSensor  OutDataTypeStr=Bus: PRESCAN_BEACONOBU_INPUT_DATA  PortDimensions=1  SampleTime=1/20  BusOutputAsStruct=on
  Actuator : S-Function  FunctionName=sfun_BeaconOBU_Input  Parameters=sensorID, timestep  EnableBusSupport=off  mask(PreScan Sink Block: RFBeacon I/O){sensorID=42, timestep=1/20}
      mask prompts: sensorID "Sensor ID"; timestep "MATLAB timestep:"
      mask help:
      | Using the Beacon and OBU (On-Board Unit) information between actors and infrastructure can be exchanged.
      |
      | The Beacon Transmitter contains the following, user-definable signals:
      |
      | - Beacon Type		[-]
      | - Spares (1:15)		[-]
      |
      | For more information, please click Help.
      mask Help: eval('openHelp(486)')
      mask Display: image(imread('ico_Beacon_RF_24_gray.png'))
  wires:
  RFBeacon_1Out/1 -> Actuator/1

== system Demo_TollSystem_cs/RFBeacon_2 ==
  Sensor : S-Function  FunctionName=sfun_Beacon  Parameters=sensorID, NrEntitiesOut, timestep  EnableBusSupport=off  mask(PreScan Source Block: RFBeacon I/O){sensorID=43, NrEntitiesOut=5, timestep=1/20}
      mask prompts: sensorID "Sensor ID"; NrEntitiesOut "User Specified: # of Visible OBUs"; timestep "MATLAB timestep:"
      mask help:
      | Using the Beacon and OBU (On-Board Unit) information between actors and infrastructure can be exchanged.
      |
      | The Beacon Receiver receives actor information and user-definable signals.
      |
      | For more information, please click Help.
      mask Help: eval('openHelp(486)')
      mask Display: image(imread('ico_Beacon_RF_24_gray.png'))
  RFBeacon_2 : Outport  Tag=outport/BeaconAndOBU/RFBeaconSensor  OutDataTypeStr=Bus: PRESCAN_BEACON_MESSAGE  PortDimensions=5  SampleTime=1/20
  wires:
  Sensor/1 -> RFBeacon_2/1

== system Demo_TollSystem_cs/RFBeacon_2Out ==
  RFBeacon_2Out : Inport  Tag=inport/BeaconAndOBU/RFBeaconSensor  OutDataTypeStr=Bus: PRESCAN_BEACONOBU_INPUT_DATA  PortDimensions=1  SampleTime=1/20  BusOutputAsStruct=on
  Actuator : S-Function  FunctionName=sfun_BeaconOBU_Input  Parameters=sensorID, timestep  EnableBusSupport=off  mask(PreScan Sink Block: RFBeacon I/O){sensorID=43, timestep=1/20}
      mask prompts: sensorID "Sensor ID"; timestep "MATLAB timestep:"
      mask help:
      | Using the Beacon and OBU (On-Board Unit) information between actors and infrastructure can be exchanged.
      |
      | The Beacon Transmitter contains the following, user-definable signals:
      |
      | - Beacon Type		[-]
      | - Spares (1:15)		[-]
      |
      | For more information, please click Help.
      mask Help: eval('openHelp(486)')
      mask Display: image(imread('ico_Beacon_RF_24_gray.png'))
  wires:
  RFBeacon_2Out/1 -> Actuator/1
